simulink model "c00002M_harness"  (R2018a)
settings: Solver=ode3  StartTime=0.0  StopTime=10.0  RelTol=1e-3  EnableMultiTasking=on
undefined symbols (not defined in the file): b, DiscIntNeverNeededParam, J, K, L, PosMinimaW3, PosMinimaW4, R, sigbuilder_block
(part 11 of 75)

== system c00002M_harness/M111 ==
  DW1 : Inport  OutMin=0  OutMax=4  OutDataTypeStr=int8
  DW2 : Inport  Port=2  OutMin=0  OutMax=4  OutDataTypeStr=int8
  DW4 : Inport  Port=3  OutMin=0  OutMax=4  OutDataTypeStr=int8
  P1W2 : Inport  Port=4  OutMin=0  OutMax=4  OutDataTypeStr=int8
  P2W3 : Inport  Port=5  OutMin=0  OutMax=4  OutDataTypeStr=int8
  P1W3 : Inport  Port=6  OutMin=0  OutMax=4  OutDataTypeStr=int8
  P3W4 : Inport  Port=7  OutMin=0  OutMax=4  OutDataTypeStr=int8
  O1 : Inport  Port=8  OutDataTypeStr=boolean
  O2 : Inport  Port=9  OutDataTypeStr=boolean
  O3 : Inport  Port=10  OutDataTypeStr=boolean
  O4 : Inport  Port=11  OutDataTypeStr=boolean
  LD : Inport  Port=12  OutDataTypeStr=boolean
  CW1C : Inport  Port=13  OutMin=0  OutMax=4  OutDataTypeStr=int8
  CW2C : Inport  Port=14  OutMin=0  OutMax=4  OutDataTypeStr=int8
  CW3C : Inport  Port=15  OutMin=0  OutMax=4  OutDataTypeStr=int8
  CW4C : Inport  Port=16  OutMin=0  OutMax=4  OutDataTypeStr=int8
  Cyber : Subsystem
  M{,1..3} (4 alike) : Memory
  Physical : Subsystem
  S1 : Subsystem
  S2 : Subsystem
  S3 : Subsystem
  S4 : Subsystem
  W1Pos : Outport
  W2Pos : Outport  Port=2
  W3Pos : Outport  Port=3
  W4Pos : Outport  Port=4
  wires:
  Cyber/4(W4) -> Physical/4(InW4)
  DW4/1 -> Cyber/7(DW4)
  Physical/4(W4) -> S4/1(PhyMeasure), W4Pos/1
  DW2/1 -> Cyber/6(DW2)
  P3W4/1 -> Cyber/11(P3W4)
  S2/1(SensorOut) -> M1/1
  Physical/2(W2) -> S2/1(PhyMeasure), W2Pos/1
  DW1/1 -> Cyber/5(DW1)
  M/1 -> Cyber/1(PosW1)
  Physical/3(W3) -> S3/1(PhyMeasure), W3Pos/1
  M1/1 -> Cyber/2(PosW2)
  S4/1(SensorOut) -> M3/1
  P1W3/1 -> Cyber/10(P1W3)
  O3/1 -> Cyber/14(OW3)
  CW1C/1 -> Cyber/17(CW1C)
  P1W2/1 -> Cyber/8(P1W2)
  M2/1 -> Cyber/3(PosW3)
  Cyber/2(W2) -> Physical/2(InW2)
  Cyber/1(W1) -> Physical/1(InW1)
  O1/1 -> Cyber/12(OW1)
  LD/1 -> Cyber/16(LD)
  Cyber/3(W3) -> Physical/3(InW3)
  O2/1 -> Cyber/13(OW2)
  S3/1(SensorOut) -> M2/1
  O4/1 -> Cyber/15(OW4)
  Physical/1(W1) -> S1/1(PhyMeasure), W1Pos/1
  CW4C/1 -> Cyber/20(CW4C)
  CW2C/1 -> Cyber/18(CW2C)
  CW3C/1 -> Cyber/19(CW3C)
  S1/1(SensorOut) -> M/1
  P2W3/1 -> Cyber/9(P2W3)
  M3/1 -> Cyber/4(PosW4)

== system c00002M_harness/M112 ==
  DW1 : Inport  OutMin=0  OutMax=4  OutDataTypeStr=int8
  DW2 : Inport  Port=2  OutMin=0  OutMax=4  OutDataTypeStr=int8
  DW4 : Inport  Port=3  OutMin=0  OutMax=4  OutDataTypeStr=int8
  P1W2 : Inport  Port=4  OutMin=0  OutMax=4  OutDataTypeStr=int8
  P2W3 : Inport  Port=5  OutMin=0  OutMax=4  OutDataTypeStr=int8
  P1W3 : Inport  Port=6  OutMin=0  OutMax=4  OutDataTypeStr=int8
  P3W4 : Inport  Port=7  OutMin=0  OutMax=4  OutDataTypeStr=int8
  O1 : Inport  Port=8  OutDataTypeStr=boolean
  O2 : Inport  Port=9  OutDataTypeStr=boolean
  O3 : Inport  Port=10  OutDataTypeStr=boolean
  O4 : Inport  Port=11  OutDataTypeStr=boolean
  LD : Inport  Port=12  OutDataTypeStr=boolean
  CW1C : Inport  Port=13  OutMin=0  OutMax=4  OutDataTypeStr=int8
  CW2C : Inport  Port=14  OutMin=0  OutMax=4  OutDataTypeStr=int8
  CW3C : Inport  Port=15  OutMin=0  OutMax=4  OutDataTypeStr=int8
  CW4C : Inport  Port=16  OutMin=0  OutMax=4  OutDataTypeStr=int8
  Cyber : Subsystem
  M{,1..3} (4 alike) : Memory
  Physical : Subsystem
  S1 : Subsystem
  S2 : Subsystem
  S3 : Subsystem
  S4 : Subsystem
  W1Pos : Outport
  W2Pos : Outport  Port=2
  W3Pos : Outport  Port=3
  W4Pos : Outport  Port=4
  wires:
  Cyber/4(W4) -> Physical/4(InW4)
  DW4/1 -> Cyber/7(DW4)
  Physical/4(W4) -> S4/1(PhyMeasure), W4Pos/1
  DW2/1 -> Cyber/6(DW2)
  P3W4/1 -> Cyber/11(P3W4)
  S2/1(SensorOut) -> M1/1
  Physical/2(W2) -> S2/1(PhyMeasure), W2Pos/1
  DW1/1 -> Cyber/5(DW1)
  M/1 -> Cyber/1(PosW1)
  Physical/3(W3) -> S3/1(PhyMeasure), W3Pos/1
  M1/1 -> Cyber/2(PosW2)
  S4/1(SensorOut) -> M3/1
  P1W3/1 -> Cyber/10(P1W3)
  O3/1 -> Cyber/14(OW3)
  CW1C/1 -> Cyber/17(CW1C)
  P1W2/1 -> Cyber/8(P1W2)
  M2/1 -> Cyber/3(PosW3)
  Cyber/2(W2) -> Physical/2(InW2)
  Cyber/1(W1) -> Physical/1(InW1)
  O1/1 -> Cyber/12(OW1)
  LD/1 -> Cyber/16(LD)
  Cyber/3(W3) -> Physical/3(InW3)
  O2/1 -> Cyber/13(OW2)
  S3/1(SensorOut) -> M2/1
  O4/1 -> Cyber/15(OW4)
  Physical/1(W1) -> S1/1(PhyMeasure), W1Pos/1
  CW4C/1 -> Cyber/20(CW4C)
  CW2C/1 -> Cyber/18(CW2C)
  CW3C/1 -> Cyber/19(CW3C)
  S1/1(SensorOut) -> M/1
  P2W3/1 -> Cyber/9(P2W3)
  M3/1 -> Cyber/4(PosW4)

== system c00002M_harness/M113 ==
  DW1 : Inport  OutMin=0  OutMax=4  OutDataTypeStr=int8
  DW2 : Inport  Port=2  OutMin=0  OutMax=4  OutDataTypeStr=int8
  DW4 : Inport  Port=3  OutMin=0  OutMax=4  OutDataTypeStr=int8
  P1W2 : Inport  Port=4  OutMin=0  OutMax=4  OutDataTypeStr=int8
  P2W3 : Inport  Port=5  OutMin=0  OutMax=4  OutDataTypeStr=int8
  P1W3 : Inport  Port=6  OutMin=0  OutMax=4  OutDataTypeStr=int8
  P3W4 : Inport  Port=7  OutMin=0  OutMax=4  OutDataTypeStr=int8
  O1 : Inport  Port=8  OutDataTypeStr=boolean
  O2 : Inport  Port=9  OutDataTypeStr=boolean
  O3 : Inport  Port=10  OutDataTypeStr=boolean
  O4 : Inport  Port=11  OutDataTypeStr=boolean
  LD : Inport  Port=12  OutDataTypeStr=boolean
  CW1C : Inport  Port=13  OutMin=0  OutMax=4  OutDataTypeStr=int8
  CW2C : Inport  Port=14  OutMin=0  OutMax=4  OutDataTypeStr=int8
  CW3C : Inport  Port=15  OutMin=0  OutMax=4  OutDataTypeStr=int8
  CW4C : Inport  Port=16  OutMin=0  OutMax=4  OutDataTypeStr=int8
  Cyber : Subsystem
  M{,1..3} (4 alike) : Memory
  Physical : Subsystem
  S1 : Subsystem
  S2 : Subsystem
  S3 : Subsystem
  S4 : Subsystem
  W1Pos : Outport
  W2Pos : Outport  Port=2
  W3Pos : Outport  Port=3
  W4Pos : Outport  Port=4
  wires:
  Cyber/4(W4) -> Physical/4(InW4)
  DW4/1 -> Cyber/7(DW4)
  Physical/4(W4) -> S4/1(PhyMeasure), W4Pos/1
  DW2/1 -> Cyber/6(DW2)
  P3W4/1 -> Cyber/11(P3W4)
  S2/1(SensorOut) -> M1/1
  Physical/2(W2) -> S2/1(PhyMeasure), W2Pos/1
  DW1/1 -> Cyber/5(DW1)
  M/1 -> Cyber/1(PosW1)
  Physical/3(W3) -> S3/1(PhyMeasure), W3Pos/1
  M1/1 -> Cyber/2(PosW2)
  S4/1(SensorOut) -> M3/1
  P1W3/1 -> Cyber/10(P1W3)
  O3/1 -> Cyber/14(OW3)
  CW1C/1 -> Cyber/17(CW1C)
  P1W2/1 -> Cyber/8(P1W2)
  M2/1 -> Cyber/3(PosW3)
  Cyber/2(W2) -> Physical/2(InW2)
  Cyber/1(W1) -> Physical/1(InW1)
  O1/1 -> Cyber/12(OW1)
  LD/1 -> Cyber/16(LD)
  Cyber/3(W3) -> Physical/3(InW3)
  O2/1 -> Cyber/13(OW2)
  S3/1(SensorOut) -> M2/1
  O4/1 -> Cyber/15(OW4)
  Physical/1(W1) -> S1/1(PhyMeasure), W1Pos/1
  CW4C/1 -> Cyber/20(CW4C)
  CW2C/1 -> Cyber/18(CW2C)
  CW3C/1 -> Cyber/19(CW3C)
  S1/1(SensorOut) -> M/1
  P2W3/1 -> Cyber/9(P2W3)
  M3/1 -> Cyber/4(PosW4)

== system c00002M_harness/M114 ==
  DW1 : Inport  OutMin=0  OutMax=4  OutDataTypeStr=int8
  DW2 : Inport  Port=2  OutMin=0  OutMax=4  OutDataTypeStr=int8
  DW4 : Inport  Port=3  OutMin=0  OutMax=4  OutDataTypeStr=int8
  P1W2 : Inport  Port=4  OutMin=0  OutMax=4  OutDataTypeStr=int8
  P2W3 : Inport  Port=5  OutMin=0  OutMax=4  OutDataTypeStr=int8
  P1W3 : Inport  Port=6  OutMin=0  OutMax=4  OutDataTypeStr=int8
  P3W4 : Inport  Port=7  OutMin=0  OutMax=4  OutDataTypeStr=int8
  O1 : Inport  Port=8  OutDataTypeStr=boolean
  O2 : Inport  Port=9  OutDataTypeStr=boolean
  O3 : Inport  Port=10  OutDataTypeStr=boolean
  O4 : Inport  Port=11  OutDataTypeStr=boolean
  LD : Inport  Port=12  OutDataTypeStr=boolean
  CW1C : Inport  Port=13  OutMin=0  OutMax=4  OutDataTypeStr=int8
  CW2C : Inport  Port=14  OutMin=0  OutMax=4  OutDataTypeStr=int8
  CW3C : Inport  Port=15  OutMin=0  OutMax=4  OutDataTypeStr=int8
  CW4C : Inport  Port=16  OutMin=0  OutMax=4  OutDataTypeStr=int8
  Cyber : Subsystem
  M{,1..3} (4 alike) : Memory
  Physical : Subsystem
  S1 : Subsystem
  S2 : Subsystem
  S3 : Subsystem
  S4 : Subsystem
  W1Pos : Outport
  W2Pos : Outport  Port=2
  W3Pos : Outport  Port=3
  W4Pos : Outport  Port=4
  wires:
  Cyber/4(W4) -> Physical/4(InW4)
  DW4/1 -> Cyber/7(DW4)
  Physical/4(W4) -> S4/1(PhyMeasure), W4Pos/1
  DW2/1 -> Cyber/6(DW2)
  P3W4/1 -> Cyber/11(P3W4)
  S2/1(SensorOut) -> M1/1
  Physical/2(W2) -> S2/1(PhyMeasure), W2Pos/1
  DW1/1 -> Cyber/5(DW1)
  M/1 -> Cyber/1(PosW1)
  Physical/3(W3) -> S3/1(PhyMeasure), W3Pos/1
  M1/1 -> Cyber/2(PosW2)
  S4/1(SensorOut) -> M3/1
  P1W3/1 -> Cyber/10(P1W3)
  O3/1 -> Cyber/14(OW3)
  CW1C/1 -> Cyber/17(CW1C)
  P1W2/1 -> Cyber/8(P1W2)
  M2/1 -> Cyber/3(PosW3)
  Cyber/2(W2) -> Physical/2(InW2)
  Cyber/1(W1) -> Physical/1(InW1)
  O1/1 -> Cyber/12(OW1)
  LD/1 -> Cyber/16(LD)
  Cyber/3(W3) -> Physical/3(InW3)
  O2/1 -> Cyber/13(OW2)
  S3/1(SensorOut) -> M2/1
  O4/1 -> Cyber/15(OW4)
  Physical/1(W1) -> S1/1(PhyMeasure), W1Pos/1
  CW4C/1 -> Cyber/20(CW4C)
  CW2C/1 -> Cyber/18(CW2C)
  CW3C/1 -> Cyber/19(CW3C)
  S1/1(SensorOut) -> M/1
  P2W3/1 -> Cyber/9(P2W3)
  M3/1 -> Cyber/4(PosW4)

== system c00002M_harness/M115 ==
  DW1 : Inport  OutMin=0  OutMax=4  OutDataTypeStr=int8
  DW2 : Inport  Port=2  OutMin=0  OutMax=4  OutDataTypeStr=int8
  DW4 : Inport  Port=3  OutMin=0  OutMax=4  OutDataTypeStr=int8
  P1W2 : Inport  Port=4  OutMin=0  OutMax=4  OutDataTypeStr=int8
  P2W3 : Inport  Port=5  OutMin=0  OutMax=4  OutDataTypeStr=int8
  P1W3 : Inport  Port=6  OutMin=0  OutMax=4  OutDataTypeStr=int8
  P3W4 : Inport  Port=7  OutMin=0  OutMax=4  OutDataTypeStr=int8
  O1 : Inport  Port=8  OutDataTypeStr=boolean
  O2 : Inport  Port=9  OutDataTypeStr=boolean
  O3 : Inport  Port=10  OutDataTypeStr=boolean
  O4 : Inport  Port=11  OutDataTypeStr=boolean
  LD : Inport  Port=12  OutDataTypeStr=boolean
  CW1C : Inport  Port=13  OutMin=0  OutMax=4  OutDataTypeStr=int8
  CW2C : Inport  Port=14  OutMin=0  OutMax=4  OutDataTypeStr=int8
  CW3C : Inport  Port=15  OutMin=0  OutMax=4  OutDataTypeStr=int8
  CW4C : Inport  Port=16  OutMin=0  OutMax=4  OutDataTypeStr=int8
  Cyber : Subsystem
  M{,1..3} (4 alike) : Memory
  Physical : Subsystem
  S1 : Subsystem
  S2 : Subsystem
  S3 : Subsystem
  S4 : Subsystem
  W1Pos : Outport
  W2Pos : Outport  Port=2
  W3Pos : Outport  Port=3
  W4Pos : Outport  Port=4
  wires:
  Cyber/4(W4) -> Physical/4(InW4)
  DW4/1 -> Cyber/7(DW4)
  Physical/4(W4) -> S4/1(PhyMeasure), W4Pos/1
  DW2/1 -> Cyber/6(DW2)
  P3W4/1 -> Cyber/11(P3W4)
  S2/1(SensorOut) -> M1/1
  Physical/2(W2) -> S2/1(PhyMeasure), W2Pos/1
  DW1/1 -> Cyber/5(DW1)
  M/1 -> Cyber/1(PosW1)
  Physical/3(W3) -> S3/1(PhyMeasure), W3Pos/1
  M1/1 -> Cyber/2(PosW2)
  S4/1(SensorOut) -> M3/1
  P1W3/1 -> Cyber/10(P1W3)
  O3/1 -> Cyber/14(OW3)
  CW1C/1 -> Cyber/17(CW1C)
  P1W2/1 -> Cyber/8(P1W2)
  M2/1 -> Cyber/3(PosW3)
  Cyber/2(W2) -> Physical/2(InW2)
  Cyber/1(W1) -> Physical/1(InW1)
  O1/1 -> Cyber/12(OW1)
  LD/1 -> Cyber/16(LD)
  Cyber/3(W3) -> Physical/3(InW3)
  O2/1 -> Cyber/13(OW2)
  S3/1(SensorOut) -> M2/1
  O4/1 -> Cyber/15(OW4)
  Physical/1(W1) -> S1/1(PhyMeasure), W1Pos/1
  CW4C/1 -> Cyber/20(CW4C)
  CW2C/1 -> Cyber/18(CW2C)
  CW3C/1 -> Cyber/19(CW3C)
  S1/1(SensorOut) -> M/1
  P2W3/1 -> Cyber/9(P2W3)
  M3/1 -> Cyber/4(PosW4)

== system c00002M_harness/M116 ==
  DW1 : Inport  OutMin=0  OutMax=4  OutDataTypeStr=int8
  DW2 : Inport  Port=2  OutMin=0  OutMax=4  OutDataTypeStr=int8
  DW4 : Inport  Port=3  OutMin=0  OutMax=4  OutDataTypeStr=int8
  P1W2 : Inport  Port=4  OutMin=0  OutMax=4  OutDataTypeStr=int8
  P2W3 : Inport  Port=5  OutMin=0  OutMax=4  OutDataTypeStr=int8
  P1W3 : Inport  Port=6  OutMin=0  OutMax=4  OutDataTypeStr=int8
  P3W4 : Inport  Port=7  OutMin=0  OutMax=4  OutDataTypeStr=int8
  O1 : Inport  Port=8  OutDataTypeStr=boolean
  O2 : Inport  Port=9  OutDataTypeStr=boolean
  O3 : Inport  Port=10  OutDataTypeStr=boolean
  O4 : Inport  Port=11  OutDataTypeStr=boolean
  LD : Inport  Port=12  OutDataTypeStr=boolean
  CW1C : Inport  Port=13  OutMin=0  OutMax=4  OutDataTypeStr=int8
  CW2C : Inport  Port=14  OutMin=0  OutMax=4  OutDataTypeStr=int8
  CW3C : Inport  Port=15  OutMin=0  OutMax=4  OutDataTypeStr=int8
  CW4C : Inport  Port=16  OutMin=0  OutMax=4  OutDataTypeStr=int8
  Cyber : Subsystem
  M{,1..3} (4 alike) : Memory
  Physical : Subsystem
  S1 : Subsystem
  S2 : Subsystem
  S3 : Subsystem
  S4 : Subsystem
  W1Pos : Outport
  W2Pos : Outport  Port=2
  W3Pos : Outport  Port=3
  W4Pos : Outport  Port=4
  wires:
  Cyber/4(W4) -> Physical/4(InW4)
  DW4/1 -> Cyber/7(DW4)
  Physical/4(W4) -> S4/1(PhyMeasure), W4Pos/1
  DW2/1 -> Cyber/6(DW2)
  P3W4/1 -> Cyber/11(P3W4)
  S2/1(SensorOut) -> M1/1
  Physical/2(W2) -> S2/1(PhyMeasure), W2Pos/1
  DW1/1 -> Cyber/5(DW1)
  M/1 -> Cyber/1(PosW1)
  Physical/3(W3) -> S3/1(PhyMeasure), W3Pos/1
  M1/1 -> Cyber/2(PosW2)
  S4/1(SensorOut) -> M3/1
  P1W3/1 -> Cyber/10(P1W3)
  O3/1 -> Cyber/14(OW3)
  CW1C/1 -> Cyber/17(CW1C)
  P1W2/1 -> Cyber/8(P1W2)
  M2/1 -> Cyber/3(PosW3)
  Cyber/2(W2) -> Physical/2(InW2)
  Cyber/1(W1) -> Physical/1(InW1)
  O1/1 -> Cyber/12(OW1)
  LD/1 -> Cyber/16(LD)
  Cyber/3(W3) -> Physical/3(InW3)
  O2/1 -> Cyber/13(OW2)
  S3/1(SensorOut) -> M2/1
  O4/1 -> Cyber/15(OW4)
  Physical/1(W1) -> S1/1(PhyMeasure), W1Pos/1
  CW4C/1 -> Cyber/20(CW4C)
  CW2C/1 -> Cyber/18(CW2C)
  CW3C/1 -> Cyber/19(CW3C)
  S1/1(SensorOut) -> M/1
  P2W3/1 -> Cyber/9(P2W3)
  M3/1 -> Cyber/4(PosW4)

== system c00002M_harness/M117 ==
  DW1 : Inport  OutMin=0  OutMax=4  OutDataTypeStr=int8
  DW2 : Inport  Port=2  OutMin=0  OutMax=4  OutDataTypeStr=int8
  DW4 : Inport  Port=3  OutMin=0  OutMax=4  OutDataTypeStr=int8
  P1W2 : Inport  Port=4  OutMin=0  OutMax=4  OutDataTypeStr=int8
  P2W3 : Inport  Port=5  OutMin=0  OutMax=4  OutDataTypeStr=int8
  P1W3 : Inport  Port=6  OutMin=0  OutMax=4  OutDataTypeStr=int8
  P3W4 : Inport  Port=7  OutMin=0  OutMax=4  OutDataTypeStr=int8
  O1 : Inport  Port=8  OutDataTypeStr=boolean
  O2 : Inport  Port=9  OutDataTypeStr=boolean
  O3 : Inport  Port=10  OutDataTypeStr=boolean
  O4 : Inport  Port=11  OutDataTypeStr=boolean
  LD : Inport  Port=12  OutDataTypeStr=boolean
  CW1C : Inport  Port=13  OutMin=0  OutMax=4  OutDataTypeStr=int8
  CW2C : Inport  Port=14  OutMin=0  OutMax=4  OutDataTypeStr=int8
  CW3C : Inport  Port=15  OutMin=0  OutMax=4  OutDataTypeStr=int8
  CW4C : Inport  Port=16  OutMin=0  OutMax=4  OutDataTypeStr=int8
  Cyber : Subsystem
  M{,1..3} (4 alike) : Memory
  Physical : Subsystem
  S1 : Subsystem
  S2 : Subsystem
  S3 : Subsystem
  S4 : Subsystem
  W1Pos : Outport
  W2Pos : Outport  Port=2
  W3Pos : Outport  Port=3
  W4Pos : Outport  Port=4
  wires:
  Cyber/4(W4) -> Physical/4(InW4)
  DW4/1 -> Cyber/7(DW4)
  Physical/4(W4) -> S4/1(PhyMeasure), W4Pos/1
  DW2/1 -> Cyber/6(DW2)
  P3W4/1 -> Cyber/11(P3W4)
  S2/1(SensorOut) -> M1/1
  Physical/2(W2) -> S2/1(PhyMeasure), W2Pos/1
  DW1/1 -> Cyber/5(DW1)
  M/1 -> Cyber/1(PosW1)
  Physical/3(W3) -> S3/1(PhyMeasure), W3Pos/1
  M1/1 -> Cyber/2(PosW2)
  S4/1(SensorOut) -> M3/1
  P1W3/1 -> Cyber/10(P1W3)
  O3/1 -> Cyber/14(OW3)
  CW1C/1 -> Cyber/17(CW1C)
  P1W2/1 -> Cyber/8(P1W2)
  M2/1 -> Cyber/3(PosW3)
  Cyber/2(W2) -> Physical/2(InW2)
  Cyber/1(W1) -> Physical/1(InW1)
  O1/1 -> Cyber/12(OW1)
  LD/1 -> Cyber/16(LD)
  Cyber/3(W3) -> Physical/3(InW3)
  O2/1 -> Cyber/13(OW2)
  S3/1(SensorOut) -> M2/1
  O4/1 -> Cyber/15(OW4)
  Physical/1(W1) -> S1/1(PhyMeasure), W1Pos/1
  CW4C/1 -> Cyber/20(CW4C)
  CW2C/1 -> Cyber/18(CW2C)
  CW3C/1 -> Cyber/19(CW3C)
  S1/1(SensorOut) -> M/1
  P2W3/1 -> Cyber/9(P2W3)
  M3/1 -> Cyber/4(PosW4)

== system c00002M_harness/M118 ==
  DW1 : Inport  OutMin=0  OutMax=4  OutDataTypeStr=int8
  DW2 : Inport  Port=2  OutMin=0  OutMax=4  OutDataTypeStr=int8
  DW4 : Inport  Port=3  OutMin=0  OutMax=4  OutDataTypeStr=int8
  P1W2 : Inport  Port=4  OutMin=0  OutMax=4  OutDataTypeStr=int8
  P2W3 : Inport  Port=5  OutMin=0  OutMax=4  OutDataTypeStr=int8
  P1W3 : Inport  Port=6  OutMin=0  OutMax=4  OutDataTypeStr=int8
  P3W4 : Inport  Port=7  OutMin=0  OutMax=4  OutDataTypeStr=int8
  O1 : Inport  Port=8  OutDataTypeStr=boolean
  O2 : Inport  Port=9  OutDataTypeStr=boolean
  O3 : Inport  Port=10  OutDataTypeStr=boolean
  O4 : Inport  Port=11  OutDataTypeStr=boolean
  LD : Inport  Port=12  OutDataTypeStr=boolean
  CW1C : Inport  Port=13  OutMin=0  OutMax=4  OutDataTypeStr=int8
  CW2C : Inport  Port=14  OutMin=0  OutMax=4  OutDataTypeStr=int8
  CW3C : Inport  Port=15  OutMin=0  OutMax=4  OutDataTypeStr=int8
  CW4C : Inport  Port=16  OutMin=0  OutMax=4  OutDataTypeStr=int8
  Cyber : Subsystem
  M{,1..3} (4 alike) : Memory
  Physical : Subsystem
  S1 : Subsystem
  S2 : Subsystem
  S3 : Subsystem
  S4 : Subsystem
  W1Pos : Outport
  W2Pos : Outport  Port=2
  W3Pos : Outport  Port=3
  W4Pos : Outport  Port=4
  wires:
  Cyber/4(W4) -> Physical/4(InW4)
  DW4/1 -> Cyber/7(DW4)
  Physical/4(W4) -> S4/1(PhyMeasure), W4Pos/1
  DW2/1 -> Cyber/6(DW2)
  P3W4/1 -> Cyber/11(P3W4)
  S2/1(SensorOut) -> M1/1
  Physical/2(W2) -> S2/1(PhyMeasure), W2Pos/1
  DW1/1 -> Cyber/5(DW1)
  M/1 -> Cyber/1(PosW1)
  Physical/3(W3) -> S3/1(PhyMeasure), W3Pos/1
  M1/1 -> Cyber/2(PosW2)
  S4/1(SensorOut) -> M3/1
  P1W3/1 -> Cyber/10(P1W3)
  O3/1 -> Cyber/14(OW3)
  CW1C/1 -> Cyber/17(CW1C)
  P1W2/1 -> Cyber/8(P1W2)
  M2/1 -> Cyber/3(PosW3)
  Cyber/2(W2) -> Physical/2(InW2)
  Cyber/1(W1) -> Physical/1(InW1)
  O1/1 -> Cyber/12(OW1)
  LD/1 -> Cyber/16(LD)
  Cyber/3(W3) -> Physical/3(InW3)
  O2/1 -> Cyber/13(OW2)
  S3/1(SensorOut) -> M2/1
  O4/1 -> Cyber/15(OW4)
  Physical/1(W1) -> S1/1(PhyMeasure), W1Pos/1
  CW4C/1 -> Cyber/20(CW4C)
  CW2C/1 -> Cyber/18(CW2C)
  CW3C/1 -> Cyber/19(CW3C)
  S1/1(SensorOut) -> M/1
  P2W3/1 -> Cyber/9(P2W3)
  M3/1 -> Cyber/4(PosW4)

== system c00002M_harness/M119 ==
  DW1 : Inport  OutMin=0  OutMax=4  OutDataTypeStr=int8
  DW2 : Inport  Port=2  OutMin=0  OutMax=4  OutDataTypeStr=int8
  DW4 : Inport  Port=3  OutMin=0  OutMax=4  OutDataTypeStr=int8
  P1W2 : Inport  Port=4  OutMin=0  OutMax=4  OutDataTypeStr=int8
  P2W3 : Inport  Port=5  OutMin=0  OutMax=4  OutDataTypeStr=int8
  P1W3 : Inport  Port=6  OutMin=0  OutMax=4  OutDataTypeStr=int8
  P3W4 : Inport  Port=7  OutMin=0  OutMax=4  OutDataTypeStr=int8
  O1 : Inport  Port=8  OutDataTypeStr=boolean
  O2 : Inport  Port=9  OutDataTypeStr=boolean
  O3 : Inport  Port=10  OutDataTypeStr=boolean
  O4 : Inport  Port=11  OutDataTypeStr=boolean
  LD : Inport  Port=12  OutDataTypeStr=boolean
  CW1C : Inport  Port=13  OutMin=0  OutMax=4  OutDataTypeStr=int8
  CW2C : Inport  Port=14  OutMin=0  OutMax=4  OutDataTypeStr=int8
  CW3C : Inport  Port=15  OutMin=0  OutMax=4  OutDataTypeStr=int8
  CW4C : Inport  Port=16  OutMin=0  OutMax=4  OutDataTypeStr=int8
  Cyber : Subsystem
  M{,1..3} (4 alike) : Memory
  Physical : Subsystem
  S1 : Subsystem
  S2 : Subsystem
  S3 : Subsystem
  S4 : Subsystem
  W1Pos : Outport
  W2Pos : Outport  Port=2
  W3Pos : Outport  Port=3
  W4Pos : Outport  Port=4
  wires:
  Cyber/4(W4) -> Physical/4(InW4)
  DW4/1 -> Cyber/7(DW4)
  Physical/4(W4) -> S4/1(PhyMeasure), W4Pos/1
  DW2/1 -> Cyber/6(DW2)
  P3W4/1 -> Cyber/11(P3W4)
  S2/1(SensorOut) -> M1/1
  Physical/2(W2) -> S2/1(PhyMeasure), W2Pos/1
  DW1/1 -> Cyber/5(DW1)
  M/1 -> Cyber/1(PosW1)
  Physical/3(W3) -> S3/1(PhyMeasure), W3Pos/1
  M1/1 -> Cyber/2(PosW2)
  S4/1(SensorOut) -> M3/1
  P1W3/1 -> Cyber/10(P1W3)
  O3/1 -> Cyber/14(OW3)
  CW1C/1 -> Cyber/17(CW1C)
  P1W2/1 -> Cyber/8(P1W2)
  M2/1 -> Cyber/3(PosW3)
  Cyber/2(W2) -> Physical/2(InW2)
  Cyber/1(W1) -> Physical/1(InW1)
  O1/1 -> Cyber/12(OW1)
  LD/1 -> Cyber/16(LD)
  Cyber/3(W3) -> Physical/3(InW3)
  O2/1 -> Cyber/13(OW2)
  S3/1(SensorOut) -> M2/1
  O4/1 -> Cyber/15(OW4)
  Physical/1(W1) -> S1/1(PhyMeasure), W1Pos/1
  CW4C/1 -> Cyber/20(CW4C)
  CW2C/1 -> Cyber/18(CW2C)
  CW3C/1 -> Cyber/19(CW3C)
  S1/1(SensorOut) -> M/1
  P2W3/1 -> Cyber/9(P2W3)
  M3/1 -> Cyber/4(PosW4)

== system c00002M_harness/M120 ==
  DW1 : Inport  OutMin=0  OutMax=4  OutDataTypeStr=int8
  DW2 : Inport  Port=2  OutMin=0  OutMax=4  OutDataTypeStr=int8
  DW4 : Inport  Port=3  OutMin=0  OutMax=4  OutDataTypeStr=int8
  P1W2 : Inport  Port=4  OutMin=0  OutMax=4  OutDataTypeStr=int8
  P2W3 : Inport  Port=5  OutMin=0  OutMax=4  OutDataTypeStr=int8
  P1W3 : Inport  Port=6  OutMin=0  OutMax=4  OutDataTypeStr=int8
  P3W4 : Inport  Port=7  OutMin=0  OutMax=4  OutDataTypeStr=int8
  O1 : Inport  Port=8  OutDataTypeStr=boolean
  O2 : Inport  Port=9  OutDataTypeStr=boolean
  O3 : Inport  Port=10  OutDataTypeStr=boolean
  O4 : Inport  Port=11  OutDataTypeStr=boolean
  LD : Inport  Port=12  OutDataTypeStr=boolean
  CW1C : Inport  Port=13  OutMin=0  OutMax=4  OutDataTypeStr=int8
  CW2C : Inport  Port=14  OutMin=0  OutMax=4  OutDataTypeStr=int8
  CW3C : Inport  Port=15  OutMin=0  OutMax=4  OutDataTypeStr=int8
  CW4C : Inport  Port=16  OutMin=0  OutMax=4  OutDataTypeStr=int8
  Cyber : Subsystem
  M{,1..3} (4 alike) : Memory
  Physical : Subsystem
  S1 : Subsystem
  S2 : Subsystem
  S3 : Subsystem
  S4 : Subsystem
  W1Pos : Outport
  W2Pos : Outport  Port=2
  W3Pos : Outport  Port=3
  W4Pos : Outport  Port=4
  wires:
  Cyber/4(W4) -> Physical/4(InW4)
  DW4/1 -> Cyber/7(DW4)
  Physical/4(W4) -> S4/1(PhyMeasure), W4Pos/1
  DW2/1 -> Cyber/6(DW2)
  P3W4/1 -> Cyber/11(P3W4)
  S2/1(SensorOut) -> M1/1
  Physical/2(W2) -> S2/1(PhyMeasure), W2Pos/1
  DW1/1 -> Cyber/5(DW1)
  M/1 -> Cyber/1(PosW1)
  Physical/3(W3) -> S3/1(PhyMeasure), W3Pos/1
  M1/1 -> Cyber/2(PosW2)
  S4/1(SensorOut) -> M3/1
  P1W3/1 -> Cyber/10(P1W3)
  O3/1 -> Cyber/14(OW3)
  CW1C/1 -> Cyber/17(CW1C)
  P1W2/1 -> Cyber/8(P1W2)
  M2/1 -> Cyber/3(PosW3)
  Cyber/2(W2) -> Physical/2(InW2)
  Cyber/1(W1) -> Physical/1(InW1)
  O1/1 -> Cyber/12(OW1)
  LD/1 -> Cyber/16(LD)
  Cyber/3(W3) -> Physical/3(InW3)
  O2/1 -> Cyber/13(OW2)
  S3/1(SensorOut) -> M2/1
  O4/1 -> Cyber/15(OW4)
  Physical/1(W1) -> S1/1(PhyMeasure), W1Pos/1
  CW4C/1 -> Cyber/20(CW4C)
  CW2C/1 -> Cyber/18(CW2C)
  CW3C/1 -> Cyber/19(CW3C)
  S1/1(SensorOut) -> M/1
  P2W3/1 -> Cyber/9(P2W3)
  M3/1 -> Cyber/4(PosW4)

== system c00002M_harness/M121 ==
  DW1 : Inport  OutMin=0  OutMax=4  OutDataTypeStr=int8
  DW2 : Inport  Port=2  OutMin=0  OutMax=4  OutDataTypeStr=int8
  DW4 : Inport  Port=3  OutMin=0  OutMax=4  OutDataTypeStr=int8
  P1W2 : Inport  Port=4  OutMin=0  OutMax=4  OutDataTypeStr=int8
  P2W3 : Inport  Port=5  OutMin=0  OutMax=4  OutDataTypeStr=int8
  P1W3 : Inport  Port=6  OutMin=0  OutMax=4  OutDataTypeStr=int8
  P3W4 : Inport  Port=7  OutMin=0  OutMax=4  OutDataTypeStr=int8
  O1 : Inport  Port=8  OutDataTypeStr=boolean
  O2 : Inport  Port=9  OutDataTypeStr=boolean
  O3 : Inport  Port=10  OutDataTypeStr=boolean
  O4 : Inport  Port=11  OutDataTypeStr=boolean
  LD : Inport  Port=12  OutDataTypeStr=boolean
  CW1C : Inport  Port=13  OutMin=0  OutMax=4  OutDataTypeStr=int8
  CW2C : Inport  Port=14  OutMin=0  OutMax=4  OutDataTypeStr=int8
  CW3C : Inport  Port=15  OutMin=0  OutMax=4  OutDataTypeStr=int8
  CW4C : Inport  Port=16  OutMin=0  OutMax=4  OutDataTypeStr=int8
  Cyber : Subsystem
  M{,1..3} (4 alike) : Memory
  Physical : Subsystem
  S1 : Subsystem
  S2 : Subsystem
  S3 : Subsystem
  S4 : Subsystem
  W1Pos : Outport
  W2Pos : Outport  Port=2
  W3Pos : Outport  Port=3
  W4Pos : Outport  Port=4
  wires:
  Cyber/4(W4) -> Physical/4(InW4)
  DW4/1 -> Cyber/7(DW4)
  Physical/4(W4) -> S4/1(PhyMeasure), W4Pos/1
  DW2/1 -> Cyber/6(DW2)
  P3W4/1 -> Cyber/11(P3W4)
  S2/1(SensorOut) -> M1/1
  Physical/2(W2) -> S2/1(PhyMeasure), W2Pos/1
  DW1/1 -> Cyber/5(DW1)
  M/1 -> Cyber/1(PosW1)
  Physical/3(W3) -> S3/1(PhyMeasure), W3Pos/1
  M1/1 -> Cyber/2(PosW2)
  S4/1(SensorOut) -> M3/1
  P1W3/1 -> Cyber/10(P1W3)
  O3/1 -> Cyber/14(OW3)
  CW1C/1 -> Cyber/17(CW1C)
  P1W2/1 -> Cyber/8(P1W2)
  M2/1 -> Cyber/3(PosW3)
  Cyber/2(W2) -> Physical/2(InW2)
  Cyber/1(W1) -> Physical/1(InW1)
  O1/1 -> Cyber/12(OW1)
  LD/1 -> Cyber/16(LD)
  Cyber/3(W3) -> Physical/3(InW3)
  O2/1 -> Cyber/13(OW2)
  S3/1(SensorOut) -> M2/1
  O4/1 -> Cyber/15(OW4)
  Physical/1(W1) -> S1/1(PhyMeasure), W1Pos/1
  CW4C/1 -> Cyber/20(CW4C)
  CW2C/1 -> Cyber/18(CW2C)
  CW3C/1 -> Cyber/19(CW3C)
  S1/1(SensorOut) -> M/1
  P2W3/1 -> Cyber/9(P2W3)
  M3/1 -> Cyber/4(PosW4)

== system c00002M_harness/M122 ==
  DW1 : Inport  OutMin=0  OutMax=4  OutDataTypeStr=int8
  DW2 : Inport  Port=2  OutMin=0  OutMax=4  OutDataTypeStr=int8
  DW4 : Inport  Port=3  OutMin=0  OutMax=4  OutDataTypeStr=int8
  P1W2 : Inport  Port=4  OutMin=0  OutMax=4  OutDataTypeStr=int8
  P2W3 : Inport  Port=5  OutMin=0  OutMax=4  OutDataTypeStr=int8
  P1W3 : Inport  Port=6  OutMin=0  OutMax=4  OutDataTypeStr=int8
  P3W4 : Inport  Port=7  OutMin=0  OutMax=4  OutDataTypeStr=int8
  O1 : Inport  Port=8  OutDataTypeStr=boolean
  O2 : Inport  Port=9  OutDataTypeStr=boolean
  O3 : Inport  Port=10  OutDataTypeStr=boolean
  O4 : Inport  Port=11  OutDataTypeStr=boolean
  LD : Inport  Port=12  OutDataTypeStr=boolean
  CW1C : Inport  Port=13  OutMin=0  OutMax=4  OutDataTypeStr=int8
  CW2C : Inport  Port=14  OutMin=0  OutMax=4  OutDataTypeStr=int8
  CW3C : Inport  Port=15  OutMin=0  OutMax=4  OutDataTypeStr=int8
  CW4C : Inport  Port=16  OutMin=0  OutMax=4  OutDataTypeStr=int8
  Cyber : Subsystem
  M{,1..3} (4 alike) : Memory
  Physical : Subsystem
  S1 : Subsystem
  S2 : Subsystem
  S3 : Subsystem
  S4 : Subsystem
  W1Pos : Outport
  W2Pos : Outport  Port=2
  W3Pos : Outport  Port=3
  W4Pos : Outport  Port=4
  wires:
  Cyber/4(W4) -> Physical/4(InW4)
  DW4/1 -> Cyber/7(DW4)
  Physical/4(W4) -> S4/1(PhyMeasure), W4Pos/1
  DW2/1 -> Cyber/6(DW2)
  P3W4/1 -> Cyber/11(P3W4)
  S2/1(SensorOut) -> M1/1
  Physical/2(W2) -> S2/1(PhyMeasure), W2Pos/1
  DW1/1 -> Cyber/5(DW1)
  M/1 -> Cyber/1(PosW1)
  Physical/3(W3) -> S3/1(PhyMeasure), W3Pos/1
  M1/1 -> Cyber/2(PosW2)
  S4/1(SensorOut) -> M3/1
  P1W3/1 -> Cyber/10(P1W3)
  O3/1 -> Cyber/14(OW3)
  CW1C/1 -> Cyber/17(CW1C)
  P1W2/1 -> Cyber/8(P1W2)
  M2/1 -> Cyber/3(PosW3)
  Cyber/2(W2) -> Physical/2(InW2)
  Cyber/1(W1) -> Physical/1(InW1)
  O1/1 -> Cyber/12(OW1)
  LD/1 -> Cyber/16(LD)
  Cyber/3(W3) -> Physical/3(InW3)
  O2/1 -> Cyber/13(OW2)
  S3/1(SensorOut) -> M2/1
  O4/1 -> Cyber/15(OW4)
  Physical/1(W1) -> S1/1(PhyMeasure), W1Pos/1
  CW4C/1 -> Cyber/20(CW4C)
  CW2C/1 -> Cyber/18(CW2C)
  CW3C/1 -> Cyber/19(CW3C)
  S1/1(SensorOut) -> M/1
  P2W3/1 -> Cyber/9(P2W3)
  M3/1 -> Cyber/4(PosW4)

== system c00002M_harness/M123 ==
  DW1 : Inport  OutMin=0  OutMax=4  OutDataTypeStr=int8
  DW2 : Inport  Port=2  OutMin=0  OutMax=4  OutDataTypeStr=int8
  DW4 : Inport  Port=3  OutMin=0  OutMax=4  OutDataTypeStr=int8
  P1W2 : Inport  Port=4  OutMin=0  OutMax=4  OutDataTypeStr=int8
  P2W3 : Inport  Port=5  OutMin=0  OutMax=4  OutDataTypeStr=int8
  P1W3 : Inport  Port=6  OutMin=0  OutMax=4  OutDataTypeStr=int8
  P3W4 : Inport  Port=7  OutMin=0  OutMax=4  OutDataTypeStr=int8
  O1 : Inport  Port=8  OutDataTypeStr=boolean
  O2 : Inport  Port=9  OutDataTypeStr=boolean
  O3 : Inport  Port=10  OutDataTypeStr=boolean
  O4 : Inport  Port=11  OutDataTypeStr=boolean
  LD : Inport  Port=12  OutDataTypeStr=boolean
  CW1C : Inport  Port=13  OutMin=0  OutMax=4  OutDataTypeStr=int8
  CW2C : Inport  Port=14  OutMin=0  OutMax=4  OutDataTypeStr=int8
  CW3C : Inport  Port=15  OutMin=0  OutMax=4  OutDataTypeStr=int8
  CW4C : Inport  Port=16  OutMin=0  OutMax=4  OutDataTypeStr=int8
  Cyber : Subsystem
  M{,1..3} (4 alike) : Memory
  Physical : Subsystem
  S1 : Subsystem
  S2 : Subsystem
  S3 : Subsystem
  S4 : Subsystem
  W1Pos : Outport
  W2Pos : Outport  Port=2
  W3Pos : Outport  Port=3
  W4Pos : Outport  Port=4
  wires:
  Cyber/4(W4) -> Physical/4(InW4)
  DW4/1 -> Cyber/7(DW4)
  Physical/4(W4) -> S4/1(PhyMeasure), W4Pos/1
  DW2/1 -> Cyber/6(DW2)
  P3W4/1 -> Cyber/11(P3W4)
  S2/1(SensorOut) -> M1/1
  Physical/2(W2) -> S2/1(PhyMeasure), W2Pos/1
  DW1/1 -> Cyber/5(DW1)
  M/1 -> Cyber/1(PosW1)
  Physical/3(W3) -> S3/1(PhyMeasure), W3Pos/1
  M1/1 -> Cyber/2(PosW2)
  S4/1(SensorOut) -> M3/1
  P1W3/1 -> Cyber/10(P1W3)
  O3/1 -> Cyber/14(OW3)
  CW1C/1 -> Cyber/17(CW1C)
  P1W2/1 -> Cyber/8(P1W2)
  M2/1 -> Cyber/3(PosW3)
  Cyber/2(W2) -> Physical/2(InW2)
  Cyber/1(W1) -> Physical/1(InW1)
  O1/1 -> Cyber/12(OW1)
  LD/1 -> Cyber/16(LD)
  Cyber/3(W3) -> Physical/3(InW3)
  O2/1 -> Cyber/13(OW2)
  S3/1(SensorOut) -> M2/1
  O4/1 -> Cyber/15(OW4)
  Physical/1(W1) -> S1/1(PhyMeasure), W1Pos/1
  CW4C/1 -> Cyber/20(CW4C)
  CW2C/1 -> Cyber/18(CW2C)
  CW3C/1 -> Cyber/19(CW3C)
  S1/1(SensorOut) -> M/1
  P2W3/1 -> Cyber/9(P2W3)
  M3/1 -> Cyber/4(PosW4)

== system c00002M_harness/M124 ==
  DW1 : Inport  OutMin=0  OutMax=4  OutDataTypeStr=int8
  DW2 : Inport  Port=2  OutMin=0  OutMax=4  OutDataTypeStr=int8
  DW4 : Inport  Port=3  OutMin=0  OutMax=4  OutDataTypeStr=int8
  P1W2 : Inport  Port=4  OutMin=0  OutMax=4  OutDataTypeStr=int8
  P2W3 : Inport  Port=5  OutMin=0  OutMax=4  OutDataTypeStr=int8
  P1W3 : Inport  Port=6  OutMin=0  OutMax=4  OutDataTypeStr=int8
  P3W4 : Inport  Port=7  OutMin=0  OutMax=4  OutDataTypeStr=int8
  O1 : Inport  Port=8  OutDataTypeStr=boolean
  O2 : Inport  Port=9  OutDataTypeStr=boolean
  O3 : Inport  Port=10  OutDataTypeStr=boolean
  O4 : Inport  Port=11  OutDataTypeStr=boolean
  LD : Inport  Port=12  OutDataTypeStr=boolean
  CW1C : Inport  Port=13  OutMin=0  OutMax=4  OutDataTypeStr=int8
  CW2C : Inport  Port=14  OutMin=0  OutMax=4  OutDataTypeStr=int8
  CW3C : Inport  Port=15  OutMin=0  OutMax=4  OutDataTypeStr=int8
  CW4C : Inport  Port=16  OutMin=0  OutMax=4  OutDataTypeStr=int8
  Cyber : Subsystem
  M{,1..3} (4 alike) : Memory
  Physical : Subsystem
  S1 : Subsystem
  S2 : Subsystem
  S3 : Subsystem
  S4 : Subsystem
  W1Pos : Outport
  W2Pos : Outport  Port=2
  W3Pos : Outport  Port=3
  W4Pos : Outport  Port=4
  wires:
  Cyber/4(W4) -> Physical/4(InW4)
  DW4/1 -> Cyber/7(DW4)
  Physical/4(W4) -> S4/1(PhyMeasure), W4Pos/1
  DW2/1 -> Cyber/6(DW2)
  P3W4/1 -> Cyber/11(P3W4)
  S2/1(SensorOut) -> M1/1
  Physical/2(W2) -> S2/1(PhyMeasure), W2Pos/1
  DW1/1 -> Cyber/5(DW1)
  M/1 -> Cyber/1(PosW1)
  Physical/3(W3) -> S3/1(PhyMeasure), W3Pos/1
  M1/1 -> Cyber/2(PosW2)
  S4/1(SensorOut) -> M3/1
  P1W3/1 -> Cyber/10(P1W3)
  O3/1 -> Cyber/14(OW3)
  CW1C/1 -> Cyber/17(CW1C)
  P1W2/1 -> Cyber/8(P1W2)
  M2/1 -> Cyber/3(PosW3)
  Cyber/2(W2) -> Physical/2(InW2)
  Cyber/1(W1) -> Physical/1(InW1)
  O1/1 -> Cyber/12(OW1)
  LD/1 -> Cyber/16(LD)
  Cyber/3(W3) -> Physical/3(InW3)
  O2/1 -> Cyber/13(OW2)
  S3/1(SensorOut) -> M2/1
  O4/1 -> Cyber/15(OW4)
  Physical/1(W1) -> S1/1(PhyMeasure), W1Pos/1
  CW4C/1 -> Cyber/20(CW4C)
  CW2C/1 -> Cyber/18(CW2C)
  CW3C/1 -> Cyber/19(CW3C)
  S1/1(SensorOut) -> M/1
  P2W3/1 -> Cyber/9(P2W3)
  M3/1 -> Cyber/4(PosW4)

== system c00002M_harness/M125 ==
  DW1 : Inport  OutMin=0  OutMax=4  OutDataTypeStr=int8
  DW2 : Inport  Port=2  OutMin=0  OutMax=4  OutDataTypeStr=int8
  DW4 : Inport  Port=3  OutMin=0  OutMax=4  OutDataTypeStr=int8
  P1W2 : Inport  Port=4  OutMin=0  OutMax=4  OutDataTypeStr=int8
  P2W3 : Inport  Port=5  OutMin=0  OutMax=4  OutDataTypeStr=int8
  P1W3 : Inport  Port=6  OutMin=0  OutMax=4  OutDataTypeStr=int8
  P3W4 : Inport  Port=7  OutMin=0  OutMax=4  OutDataTypeStr=int8
  O1 : Inport  Port=8  OutDataTypeStr=boolean
  O2 : Inport  Port=9  OutDataTypeStr=boolean
  O3 : Inport  Port=10  OutDataTypeStr=boolean
  O4 : Inport  Port=11  OutDataTypeStr=boolean
  LD : Inport  Port=12  OutDataTypeStr=boolean
  CW1C : Inport  Port=13  OutMin=0  OutMax=4  OutDataTypeStr=int8
  CW2C : Inport  Port=14  OutMin=0  OutMax=4  OutDataTypeStr=int8
  CW3C : Inport  Port=15  OutMin=0  OutMax=4  OutDataTypeStr=int8
  CW4C : Inport  Port=16  OutMin=0  OutMax=4  OutDataTypeStr=int8
  Cyber : Subsystem
  M{,1..3} (4 alike) : Memory
  Physical : Subsystem
  S1 : Subsystem
  S2 : Subsystem
  S3 : Subsystem
  S4 : Subsystem
  W1Pos : Outport
  W2Pos : Outport  Port=2
  W3Pos : Outport  Port=3
  W4Pos : Outport  Port=4
  wires:
  Cyber/4(W4) -> Physical/4(InW4)
  DW4/1 -> Cyber/7(DW4)
  Physical/4(W4) -> S4/1(PhyMeasure), W4Pos/1
  DW2/1 -> Cyber/6(DW2)
  P3W4/1 -> Cyber/11(P3W4)
  S2/1(SensorOut) -> M1/1
  Physical/2(W2) -> S2/1(PhyMeasure), W2Pos/1
  DW1/1 -> Cyber/5(DW1)
  M/1 -> Cyber/1(PosW1)
  Physical/3(W3) -> S3/1(PhyMeasure), W3Pos/1
  M1/1 -> Cyber/2(PosW2)
  S4/1(SensorOut) -> M3/1
  P1W3/1 -> Cyber/10(P1W3)
  O3/1 -> Cyber/14(OW3)
  CW1C/1 -> Cyber/17(CW1C)
  P1W2/1 -> Cyber/8(P1W2)
  M2/1 -> Cyber/3(PosW3)
  Cyber/2(W2) -> Physical/2(InW2)
  Cyber/1(W1) -> Physical/1(InW1)
  O1/1 -> Cyber/12(OW1)
  LD/1 -> Cyber/16(LD)
  Cyber/3(W3) -> Physical/3(InW3)
  O2/1 -> Cyber/13(OW2)
  S3/1(SensorOut) -> M2/1
  O4/1 -> Cyber/15(OW4)
  Physical/1(W1) -> S1/1(PhyMeasure), W1Pos/1
  CW4C/1 -> Cyber/20(CW4C)
  CW2C/1 -> Cyber/18(CW2C)
  CW3C/1 -> Cyber/19(CW3C)
  S1/1(SensorOut) -> M/1
  P2W3/1 -> Cyber/9(P2W3)
  M3/1 -> Cyber/4(PosW4)

== system c00002M_harness/M126 ==
  DW1 : Inport  OutMin=0  OutMax=4  OutDataTypeStr=int8
  DW2 : Inport  Port=2  OutMin=0  OutMax=4  OutDataTypeStr=int8
  DW4 : Inport  Port=3  OutMin=0  OutMax=4  OutDataTypeStr=int8
  P1W2 : Inport  Port=4  OutMin=0  OutMax=4  OutDataTypeStr=int8
  P2W3 : Inport  Port=5  OutMin=0  OutMax=4  OutDataTypeStr=int8
  P1W3 : Inport  Port=6  OutMin=0  OutMax=4  OutDataTypeStr=int8
  P3W4 : Inport  Port=7  OutMin=0  OutMax=4  OutDataTypeStr=int8
  O1 : Inport  Port=8  OutDataTypeStr=boolean
  O2 : Inport  Port=9  OutDataTypeStr=boolean
  O3 : Inport  Port=10  OutDataTypeStr=boolean
  O4 : Inport  Port=11  OutDataTypeStr=boolean
  LD : Inport  Port=12  OutDataTypeStr=boolean
  CW1C : Inport  Port=13  OutMin=0  OutMax=4  OutDataTypeStr=int8
  CW2C : Inport  Port=14  OutMin=0  OutMax=4  OutDataTypeStr=int8
  CW3C : Inport  Port=15  OutMin=0  OutMax=4  OutDataTypeStr=int8
  CW4C : Inport  Port=16  OutMin=0  OutMax=4  OutDataTypeStr=int8
  Cyber : Subsystem
  M{,1..3} (4 alike) : Memory
  Physical : Subsystem
  S1 : Subsystem
  S2 : Subsystem
  S3 : Subsystem
  S4 : Subsystem
  W1Pos : Outport
  W2Pos : Outport  Port=2
  W3Pos : Outport  Port=3
  W4Pos : Outport  Port=4
  wires:
  Cyber/4(W4) -> Physical/4(InW4)
  DW4/1 -> Cyber/7(DW4)
  Physical/4(W4) -> S4/1(PhyMeasure), W4Pos/1
  DW2/1 -> Cyber/6(DW2)
  P3W4/1 -> Cyber/11(P3W4)
  S2/1(SensorOut) -> M1/1
  Physical/2(W2) -> S2/1(PhyMeasure), W2Pos/1
  DW1/1 -> Cyber/5(DW1)
  M/1 -> Cyber/1(PosW1)
  Physical/3(W3) -> S3/1(PhyMeasure), W3Pos/1
  M1/1 -> Cyber/2(PosW2)
  S4/1(SensorOut) -> M3/1
  P1W3/1 -> Cyber/10(P1W3)
  O3/1 -> Cyber/14(OW3)
  CW1C/1 -> Cyber/17(CW1C)
  P1W2/1 -> Cyber/8(P1W2)
  M2/1 -> Cyber/3(PosW3)
  Cyber/2(W2) -> Physical/2(InW2)
  Cyber/1(W1) -> Physical/1(InW1)
  O1/1 -> Cyber/12(OW1)
  LD/1 -> Cyber/16(LD)
  Cyber/3(W3) -> Physical/3(InW3)
  O2/1 -> Cyber/13(OW2)
  S3/1(SensorOut) -> M2/1
  O4/1 -> Cyber/15(OW4)
  Physical/1(W1) -> S1/1(PhyMeasure), W1Pos/1
  CW4C/1 -> Cyber/20(CW4C)
  CW2C/1 -> Cyber/18(CW2C)
  CW3C/1 -> Cyber/19(CW3C)
  S1/1(SensorOut) -> M/1
  P2W3/1 -> Cyber/9(P2W3)
  M3/1 -> Cyber/4(PosW4)

== system c00002M_harness/M127 ==
  DW1 : Inport  OutMin=0  OutMax=4  OutDataTypeStr=int8
  DW2 : Inport  Port=2  OutMin=0  OutMax=4  OutDataTypeStr=int8
  DW4 : Inport  Port=3  OutMin=0  OutMax=4  OutDataTypeStr=int8
  P1W2 : Inport  Port=4  OutMin=0  OutMax=4  OutDataTypeStr=int8
  P2W3 : Inport  Port=5  OutMin=0  OutMax=4  OutDataTypeStr=int8
  P1W3 : Inport  Port=6  OutMin=0  OutMax=4  OutDataTypeStr=int8
  P3W4 : Inport  Port=7  OutMin=0  OutMax=4  OutDataTypeStr=int8
  O1 : Inport  Port=8  OutDataTypeStr=boolean
  O2 : Inport  Port=9  OutDataTypeStr=boolean
  O3 : Inport  Port=10  OutDataTypeStr=boolean
  O4 : Inport  Port=11  OutDataTypeStr=boolean
  LD : Inport  Port=12  OutDataTypeStr=boolean
  CW1C : Inport  Port=13  OutMin=0  OutMax=4  OutDataTypeStr=int8
  CW2C : Inport  Port=14  OutMin=0  OutMax=4  OutDataTypeStr=int8
  CW3C : Inport  Port=15  OutMin=0  OutMax=4  OutDataTypeStr=int8
  CW4C : Inport  Port=16  OutMin=0  OutMax=4  OutDataTypeStr=int8
  Cyber : Subsystem
  M{,1..3} (4 alike) : Memory
  Physical : Subsystem
  S1 : Subsystem
  S2 : Subsystem
  S3 : Subsystem
  S4 : Subsystem
  W1Pos : Outport
  W2Pos : Outport  Port=2
  W3Pos : Outport  Port=3
  W4Pos : Outport  Port=4
  wires:
  Cyber/4(W4) -> Physical/4(InW4)
  DW4/1 -> Cyber/7(DW4)
  Physical/4(W4) -> S4/1(PhyMeasure), W4Pos/1
  DW2/1 -> Cyber/6(DW2)
  P3W4/1 -> Cyber/11(P3W4)
  S2/1(SensorOut) -> M1/1
  Physical/2(W2) -> S2/1(PhyMeasure), W2Pos/1
  DW1/1 -> Cyber/5(DW1)
  M/1 -> Cyber/1(PosW1)
  Physical/3(W3) -> S3/1(PhyMeasure), W3Pos/1
  M1/1 -> Cyber/2(PosW2)
  S4/1(SensorOut) -> M3/1
  P1W3/1 -> Cyber/10(P1W3)
  O3/1 -> Cyber/14(OW3)
  CW1C/1 -> Cyber/17(CW1C)
  P1W2/1 -> Cyber/8(P1W2)
  M2/1 -> Cyber/3(PosW3)
  Cyber/2(W2) -> Physical/2(InW2)
  Cyber/1(W1) -> Physical/1(InW1)
  O1/1 -> Cyber/12(OW1)
  LD/1 -> Cyber/16(LD)
  Cyber/3(W3) -> Physical/3(InW3)
  O2/1 -> Cyber/13(OW2)
  S3/1(SensorOut) -> M2/1
  O4/1 -> Cyber/15(OW4)
  Physical/1(W1) -> S1/1(PhyMeasure), W1Pos/1
  CW4C/1 -> Cyber/20(CW4C)
  CW2C/1 -> Cyber/18(CW2C)
  CW3C/1 -> Cyber/19(CW3C)
  S1/1(SensorOut) -> M/1
  P2W3/1 -> Cyber/9(P2W3)
  M3/1 -> Cyber/4(PosW4)

== system c00002M_harness/M128 ==
  DW1 : Inport  OutMin=0  OutMax=4  OutDataTypeStr=int8
  DW2 : Inport  Port=2  OutMin=0  OutMax=4  OutDataTypeStr=int8
  DW4 : Inport  Port=3  OutMin=0  OutMax=4  OutDataTypeStr=int8
  P1W2 : Inport  Port=4  OutMin=0  OutMax=4  OutDataTypeStr=int8
  P2W3 : Inport  Port=5  OutMin=0  OutMax=4  OutDataTypeStr=int8
  P1W3 : Inport  Port=6  OutMin=0  OutMax=4  OutDataTypeStr=int8
  P3W4 : Inport  Port=7  OutMin=0  OutMax=4  OutDataTypeStr=int8
  O1 : Inport  Port=8  OutDataTypeStr=boolean
  O2 : Inport  Port=9  OutDataTypeStr=boolean
  O3 : Inport  Port=10  OutDataTypeStr=boolean
  O4 : Inport  Port=11  OutDataTypeStr=boolean
  LD : Inport  Port=12  OutDataTypeStr=boolean
  CW1C : Inport  Port=13  OutMin=0  OutMax=4  OutDataTypeStr=int8
  CW2C : Inport  Port=14  OutMin=0  OutMax=4  OutDataTypeStr=int8
  CW3C : Inport  Port=15  OutMin=0  OutMax=4  OutDataTypeStr=int8
  CW4C : Inport  Port=16  OutMin=0  OutMax=4  OutDataTypeStr=int8
  Cyber : Subsystem
  M{,1..3} (4 alike) : Memory
  Physical : Subsystem
  S1 : Subsystem
  S2 : Subsystem
  S3 : Subsystem
  S4 : Subsystem
  W1Pos : Outport
  W2Pos : Outport  Port=2
  W3Pos : Outport  Port=3
  W4Pos : Outport  Port=4
  wires:
  Cyber/4(W4) -> Physical/4(InW4)
  DW4/1 -> Cyber/7(DW4)
  Physical/4(W4) -> S4/1(PhyMeasure), W4Pos/1
  DW2/1 -> Cyber/6(DW2)
  P3W4/1 -> Cyber/11(P3W4)
  S2/1(SensorOut) -> M1/1
  Physical/2(W2) -> S2/1(PhyMeasure), W2Pos/1
  DW1/1 -> Cyber/5(DW1)
  M/1 -> Cyber/1(PosW1)
  Physical/3(W3) -> S3/1(PhyMeasure), W3Pos/1
  M1/1 -> Cyber/2(PosW2)
  S4/1(SensorOut) -> M3/1
  P1W3/1 -> Cyber/10(P1W3)
  O3/1 -> Cyber/14(OW3)
  CW1C/1 -> Cyber/17(CW1C)
  P1W2/1 -> Cyber/8(P1W2)
  M2/1 -> Cyber/3(PosW3)
  Cyber/2(W2) -> Physical/2(InW2)
  Cyber/1(W1) -> Physical/1(InW1)
  O1/1 -> Cyber/12(OW1)
  LD/1 -> Cyber/16(LD)
  Cyber/3(W3) -> Physical/3(InW3)
  O2/1 -> Cyber/13(OW2)
  S3/1(SensorOut) -> M2/1
  O4/1 -> Cyber/15(OW4)
  Physical/1(W1) -> S1/1(PhyMeasure), W1Pos/1
  CW4C/1 -> Cyber/20(CW4C)
  CW2C/1 -> Cyber/18(CW2C)
  CW3C/1 -> Cyber/19(CW3C)
  S1/1(SensorOut) -> M/1
  P2W3/1 -> Cyber/9(P2W3)
  M3/1 -> Cyber/4(PosW4)

== system c00002M_harness/M129 ==
  DW1 : Inport  OutMin=0  OutMax=4  OutDataTypeStr=int8
  DW2 : Inport  Port=2  OutMin=0  OutMax=4  OutDataTypeStr=int8
  DW4 : Inport  Port=3  OutMin=0  OutMax=4  OutDataTypeStr=int8
  P1W2 : Inport  Port=4  OutMin=0  OutMax=4  OutDataTypeStr=int8
  P2W3 : Inport  Port=5  OutMin=0  OutMax=4  OutDataTypeStr=int8
  P1W3 : Inport  Port=6  OutMin=0  OutMax=4  OutDataTypeStr=int8
  P3W4 : Inport  Port=7  OutMin=0  OutMax=4  OutDataTypeStr=int8
  O1 : Inport  Port=8  OutDataTypeStr=boolean
  O2 : Inport  Port=9  OutDataTypeStr=boolean
  O3 : Inport  Port=10  OutDataTypeStr=boolean
  O4 : Inport  Port=11  OutDataTypeStr=boolean
  LD : Inport  Port=12  OutDataTypeStr=boolean
  CW1C : Inport  Port=13  OutMin=0  OutMax=4  OutDataTypeStr=int8
  CW2C : Inport  Port=14  OutMin=0  OutMax=4  OutDataTypeStr=int8
  CW3C : Inport  Port=15  OutMin=0  OutMax=4  OutDataTypeStr=int8
  CW4C : Inport  Port=16  OutMin=0  OutMax=4  OutDataTypeStr=int8
  Cyber : Subsystem
  M{,1..3} (4 alike) : Memory
  Physical : Subsystem
  S1 : Subsystem
  S2 : Subsystem
  S3 : Subsystem
  S4 : Subsystem
  W1Pos : Outport
  W2Pos : Outport  Port=2
  W3Pos : Outport  Port=3
  W4Pos : Outport  Port=4
  wires:
  Cyber/4(W4) -> Physical/4(InW4)
  DW4/1 -> Cyber/7(DW4)
  Physical/4(W4) -> S4/1(PhyMeasure), W4Pos/1
  DW2/1 -> Cyber/6(DW2)
  P3W4/1 -> Cyber/11(P3W4)
  S2/1(SensorOut) -> M1/1
  Physical/2(W2) -> S2/1(PhyMeasure), W2Pos/1
  DW1/1 -> Cyber/5(DW1)
  M/1 -> Cyber/1(PosW1)
  Physical/3(W3) -> S3/1(PhyMeasure), W3Pos/1
  M1/1 -> Cyber/2(PosW2)
  S4/1(SensorOut) -> M3/1
  P1W3/1 -> Cyber/10(P1W3)
  O3/1 -> Cyber/14(OW3)
  CW1C/1 -> Cyber/17(CW1C)
  P1W2/1 -> Cyber/8(P1W2)
  M2/1 -> Cyber/3(PosW3)
  Cyber/2(W2) -> Physical/2(InW2)
  Cyber/1(W1) -> Physical/1(InW1)
  O1/1 -> Cyber/12(OW1)
  LD/1 -> Cyber/16(LD)
  Cyber/3(W3) -> Physical/3(InW3)
  O2/1 -> Cyber/13(OW2)
  S3/1(SensorOut) -> M2/1
  O4/1 -> Cyber/15(OW4)
  Physical/1(W1) -> S1/1(PhyMeasure), W1Pos/1
  CW4C/1 -> Cyber/20(CW4C)
  CW2C/1 -> Cyber/18(CW2C)
  CW3C/1 -> Cyber/19(CW3C)
  S1/1(SensorOut) -> M/1
  P2W3/1 -> Cyber/9(P2W3)
  M3/1 -> Cyber/4(PosW4)

== system c00002M_harness/M130 ==
  DW1 : Inport  OutMin=0  OutMax=4  OutDataTypeStr=int8
  DW2 : Inport  Port=2  OutMin=0  OutMax=4  OutDataTypeStr=int8
  DW4 : Inport  Port=3  OutMin=0  OutMax=4  OutDataTypeStr=int8
  P1W2 : Inport  Port=4  OutMin=0  OutMax=4  OutDataTypeStr=int8
  P2W3 : Inport  Port=5  OutMin=0  OutMax=4  OutDataTypeStr=int8
  P1W3 : Inport  Port=6  OutMin=0  OutMax=4  OutDataTypeStr=int8
  P3W4 : Inport  Port=7  OutMin=0  OutMax=4  OutDataTypeStr=int8
  O1 : Inport  Port=8  OutDataTypeStr=boolean
  O2 : Inport  Port=9  OutDataTypeStr=boolean
  O3 : Inport  Port=10  OutDataTypeStr=boolean
  O4 : Inport  Port=11  OutDataTypeStr=boolean
  LD : Inport  Port=12  OutDataTypeStr=boolean
  CW1C : Inport  Port=13  OutMin=0  OutMax=4  OutDataTypeStr=int8
  CW2C : Inport  Port=14  OutMin=0  OutMax=4  OutDataTypeStr=int8
  CW3C : Inport  Port=15  OutMin=0  OutMax=4  OutDataTypeStr=int8
  CW4C : Inport  Port=16  OutMin=0  OutMax=4  OutDataTypeStr=int8
  Cyber : Subsystem
  M{,1..3} (4 alike) : Memory
  Physical : Subsystem
  S1 : Subsystem
  S2 : Subsystem
  S3 : Subsystem
  S4 : Subsystem
  W1Pos : Outport
  W2Pos : Outport  Port=2
  W3Pos : Outport  Port=3
  W4Pos : Outport  Port=4
  wires:
  Cyber/4(W4) -> Physical/4(InW4)
  DW4/1 -> Cyber/7(DW4)
  Physical/4(W4) -> S4/1(PhyMeasure), W4Pos/1
  DW2/1 -> Cyber/6(DW2)
  P3W4/1 -> Cyber/11(P3W4)
  S2/1(SensorOut) -> M1/1
  Physical/2(W2) -> S2/1(PhyMeasure), W2Pos/1
  DW1/1 -> Cyber/5(DW1)
  M/1 -> Cyber/1(PosW1)
  Physical/3(W3) -> S3/1(PhyMeasure), W3Pos/1
  M1/1 -> Cyber/2(PosW2)
  S4/1(SensorOut) -> M3/1
  P1W3/1 -> Cyber/10(P1W3)
  O3/1 -> Cyber/14(OW3)
  CW1C/1 -> Cyber/17(CW1C)
  P1W2/1 -> Cyber/8(P1W2)
  M2/1 -> Cyber/3(PosW3)
  Cyber/2(W2) -> Physical/2(InW2)
  Cyber/1(W1) -> Physical/1(InW1)
  O1/1 -> Cyber/12(OW1)
  LD/1 -> Cyber/16(LD)
  Cyber/3(W3) -> Physical/3(InW3)
  O2/1 -> Cyber/13(OW2)
  S3/1(SensorOut) -> M2/1
  O4/1 -> Cyber/15(OW4)
  Physical/1(W1) -> S1/1(PhyMeasure), W1Pos/1
  CW4C/1 -> Cyber/20(CW4C)
  CW2C/1 -> Cyber/18(CW2C)
  CW3C/1 -> Cyber/19(CW3C)
  S1/1(SensorOut) -> M/1
  P2W3/1 -> Cyber/9(P2W3)
  M3/1 -> Cyber/4(PosW4)

== system c00002M_harness/M131 ==
  DW1 : Inport  OutMin=0  OutMax=4  OutDataTypeStr=int8
  DW2 : Inport  Port=2  OutMin=0  OutMax=4  OutDataTypeStr=int8
  DW4 : Inport  Port=3  OutMin=0  OutMax=4  OutDataTypeStr=int8
  P1W2 : Inport  Port=4  OutMin=0  OutMax=4  OutDataTypeStr=int8
  P2W3 : Inport  Port=5  OutMin=0  OutMax=4  OutDataTypeStr=int8
  P1W3 : Inport  Port=6  OutMin=0  OutMax=4  OutDataTypeStr=int8
  P3W4 : Inport  Port=7  OutMin=0  OutMax=4  OutDataTypeStr=int8
  O1 : Inport  Port=8  OutDataTypeStr=boolean
  O2 : Inport  Port=9  OutDataTypeStr=boolean
  O3 : Inport  Port=10  OutDataTypeStr=boolean
  O4 : Inport  Port=11  OutDataTypeStr=boolean
  LD : Inport  Port=12  OutDataTypeStr=boolean
  CW1C : Inport  Port=13  OutMin=0  OutMax=4  OutDataTypeStr=int8
  CW2C : Inport  Port=14  OutMin=0  OutMax=4  OutDataTypeStr=int8
  CW3C : Inport  Port=15  OutMin=0  OutMax=4  OutDataTypeStr=int8
  CW4C : Inport  Port=16  OutMin=0  OutMax=4  OutDataTypeStr=int8
  Cyber : Subsystem
  M{,1..3} (4 alike) : Memory
  Physical : Subsystem
  S1 : Subsystem
  S2 : Subsystem
  S3 : Subsystem
  S4 : Subsystem
  W1Pos : Outport
  W2Pos : Outport  Port=2
  W3Pos : Outport  Port=3
  W4Pos : Outport  Port=4
  wires:
  Cyber/4(W4) -> Physical/4(InW4)
  DW4/1 -> Cyber/7(DW4)
  Physical/4(W4) -> S4/1(PhyMeasure), W4Pos/1
  DW2/1 -> Cyber/6(DW2)
  P3W4/1 -> Cyber/11(P3W4)
  S2/1(SensorOut) -> M1/1
  Physical/2(W2) -> S2/1(PhyMeasure), W2Pos/1
  DW1/1 -> Cyber/5(DW1)
  M/1 -> Cyber/1(PosW1)
  Physical/3(W3) -> S3/1(PhyMeasure), W3Pos/1
  M1/1 -> Cyber/2(PosW2)
  S4/1(SensorOut) -> M3/1
  P1W3/1 -> Cyber/10(P1W3)
  O3/1 -> Cyber/14(OW3)
  CW1C/1 -> Cyber/17(CW1C)
  P1W2/1 -> Cyber/8(P1W2)
  M2/1 -> Cyber/3(PosW3)
  Cyber/2(W2) -> Physical/2(InW2)
  Cyber/1(W1) -> Physical/1(InW1)
  O1/1 -> Cyber/12(OW1)
  LD/1 -> Cyber/16(LD)
  Cyber/3(W3) -> Physical/3(InW3)
  O2/1 -> Cyber/13(OW2)
  S3/1(SensorOut) -> M2/1
  O4/1 -> Cyber/15(OW4)
  Physical/1(W1) -> S1/1(PhyMeasure), W1Pos/1
  CW4C/1 -> Cyber/20(CW4C)
  CW2C/1 -> Cyber/18(CW2C)
  CW3C/1 -> Cyber/19(CW3C)
  S1/1(SensorOut) -> M/1
  P2W3/1 -> Cyber/9(P2W3)
  M3/1 -> Cyber/4(PosW4)

== system c00002M_harness/M132 ==
  DW1 : Inport  OutMin=0  OutMax=4  OutDataTypeStr=int8
  DW2 : Inport  Port=2  OutMin=0  OutMax=4  OutDataTypeStr=int8
  DW4 : Inport  Port=3  OutMin=0  OutMax=4  OutDataTypeStr=int8
  P1W2 : Inport  Port=4  OutMin=0  OutMax=4  OutDataTypeStr=int8
  P2W3 : Inport  Port=5  OutMin=0  OutMax=4  OutDataTypeStr=int8
  P1W3 : Inport  Port=6  OutMin=0  OutMax=4  OutDataTypeStr=int8
  P3W4 : Inport  Port=7  OutMin=0  OutMax=4  OutDataTypeStr=int8
  O1 : Inport  Port=8  OutDataTypeStr=boolean
  O2 : Inport  Port=9  OutDataTypeStr=boolean
  O3 : Inport  Port=10  OutDataTypeStr=boolean
  O4 : Inport  Port=11  OutDataTypeStr=boolean
  LD : Inport  Port=12  OutDataTypeStr=boolean
  CW1C : Inport  Port=13  OutMin=0  OutMax=4  OutDataTypeStr=int8
  CW2C : Inport  Port=14  OutMin=0  OutMax=4  OutDataTypeStr=int8
  CW3C : Inport  Port=15  OutMin=0  OutMax=4  OutDataTypeStr=int8
  CW4C : Inport  Port=16  OutMin=0  OutMax=4  OutDataTypeStr=int8
  Cyber : Subsystem
  M{,1..3} (4 alike) : Memory
  Physical : Subsystem
  S1 : Subsystem
  S2 : Subsystem
  S3 : Subsystem
  S4 : Subsystem
  W1Pos : Outport
  W2Pos : Outport  Port=2
  W3Pos : Outport  Port=3
  W4Pos : Outport  Port=4
  wires:
  Cyber/4(W4) -> Physical/4(InW4)
  DW4/1 -> Cyber/7(DW4)
  Physical/4(W4) -> S4/1(PhyMeasure), W4Pos/1
  DW2/1 -> Cyber/6(DW2)
  P3W4/1 -> Cyber/11(P3W4)
  S2/1(SensorOut) -> M1/1
  Physical/2(W2) -> S2/1(PhyMeasure), W2Pos/1
  DW1/1 -> Cyber/5(DW1)
  M/1 -> Cyber/1(PosW1)
  Physical/3(W3) -> S3/1(PhyMeasure), W3Pos/1
  M1/1 -> Cyber/2(PosW2)
  S4/1(SensorOut) -> M3/1
  P1W3/1 -> Cyber/10(P1W3)
  O3/1 -> Cyber/14(OW3)
  CW1C/1 -> Cyber/17(CW1C)
  P1W2/1 -> Cyber/8(P1W2)
  M2/1 -> Cyber/3(PosW3)
  Cyber/2(W2) -> Physical/2(InW2)
  Cyber/1(W1) -> Physical/1(InW1)
  O1/1 -> Cyber/12(OW1)
  LD/1 -> Cyber/16(LD)
  Cyber/3(W3) -> Physical/3(InW3)
  O2/1 -> Cyber/13(OW2)
  S3/1(SensorOut) -> M2/1
  O4/1 -> Cyber/15(OW4)
  Physical/1(W1) -> S1/1(PhyMeasure), W1Pos/1
  CW4C/1 -> Cyber/20(CW4C)
  CW2C/1 -> Cyber/18(CW2C)
  CW3C/1 -> Cyber/19(CW3C)
  S1/1(SensorOut) -> M/1
  P2W3/1 -> Cyber/9(P2W3)
  M3/1 -> Cyber/4(PosW4)

== system c00002M_harness/M133 ==
  DW1 : Inport  OutMin=0  OutMax=4  OutDataTypeStr=int8
  DW2 : Inport  Port=2  OutMin=0  OutMax=4  OutDataTypeStr=int8
  DW4 : Inport  Port=3  OutMin=0  OutMax=4  OutDataTypeStr=int8
  P1W2 : Inport  Port=4  OutMin=0  OutMax=4  OutDataTypeStr=int8
  P2W3 : Inport  Port=5  OutMin=0  OutMax=4  OutDataTypeStr=int8
  P1W3 : Inport  Port=6  OutMin=0  OutMax=4  OutDataTypeStr=int8
  P3W4 : Inport  Port=7  OutMin=0  OutMax=4  OutDataTypeStr=int8
  O1 : Inport  Port=8  OutDataTypeStr=boolean
  O2 : Inport  Port=9  OutDataTypeStr=boolean
  O3 : Inport  Port=10  OutDataTypeStr=boolean
  O4 : Inport  Port=11  OutDataTypeStr=boolean
  LD : Inport  Port=12  OutDataTypeStr=boolean
  CW1C : Inport  Port=13  OutMin=0  OutMax=4  OutDataTypeStr=int8
  CW2C : Inport  Port=14  OutMin=0  OutMax=4  OutDataTypeStr=int8
  CW3C : Inport  Port=15  OutMin=0  OutMax=4  OutDataTypeStr=int8
  CW4C : Inport  Port=16  OutMin=0  OutMax=4  OutDataTypeStr=int8
  Cyber : Subsystem
  M{,1..3} (4 alike) : Memory
  Physical : Subsystem
  S1 : Subsystem
  S2 : Subsystem
  S3 : Subsystem
  S4 : Subsystem
  W1Pos : Outport
  W2Pos : Outport  Port=2
  W3Pos : Outport  Port=3
  W4Pos : Outport  Port=4
  wires:
  Cyber/4(W4) -> Physical/4(InW4)
  DW4/1 -> Cyber/7(DW4)
  Physical/4(W4) -> S4/1(PhyMeasure), W4Pos/1
  DW2/1 -> Cyber/6(DW2)
  P3W4/1 -> Cyber/11(P3W4)
  S2/1(SensorOut) -> M1/1
  Physical/2(W2) -> S2/1(PhyMeasure), W2Pos/1
  DW1/1 -> Cyber/5(DW1)
  M/1 -> Cyber/1(PosW1)
  Physical/3(W3) -> S3/1(PhyMeasure), W3Pos/1
  M1/1 -> Cyber/2(PosW2)
  S4/1(SensorOut) -> M3/1
  P1W3/1 -> Cyber/10(P1W3)
  O3/1 -> Cyber/14(OW3)
  CW1C/1 -> Cyber/17(CW1C)
  P1W2/1 -> Cyber/8(P1W2)
  M2/1 -> Cyber/3(PosW3)
  Cyber/2(W2) -> Physical/2(InW2)
  Cyber/1(W1) -> Physical/1(InW1)
  O1/1 -> Cyber/12(OW1)
  LD/1 -> Cyber/16(LD)
  Cyber/3(W3) -> Physical/3(InW3)
  O2/1 -> Cyber/13(OW2)
  S3/1(SensorOut) -> M2/1
  O4/1 -> Cyber/15(OW4)
  Physical/1(W1) -> S1/1(PhyMeasure), W1Pos/1
  CW4C/1 -> Cyber/20(CW4C)
  CW2C/1 -> Cyber/18(CW2C)
  CW3C/1 -> Cyber/19(CW3C)
  S1/1(SensorOut) -> M/1
  P2W3/1 -> Cyber/9(P2W3)
  M3/1 -> Cyber/4(PosW4)
